simulink model "sampleModel1497"  (R2023a)
settings: Solver=VariableStepAuto  StartTime=0.0  StopTime=10.0  RelTol=1e-3
libraries: hdlsllib x5, simulink x2
settings Model: Creator=user1  LastModifiedBy=user1

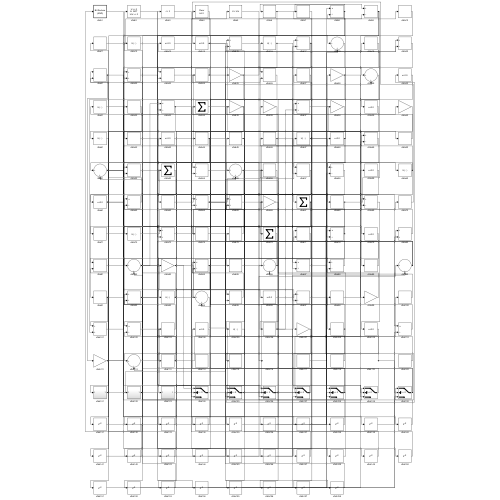
[thumbnail: Simulink's stored preview of the top-level diagram]
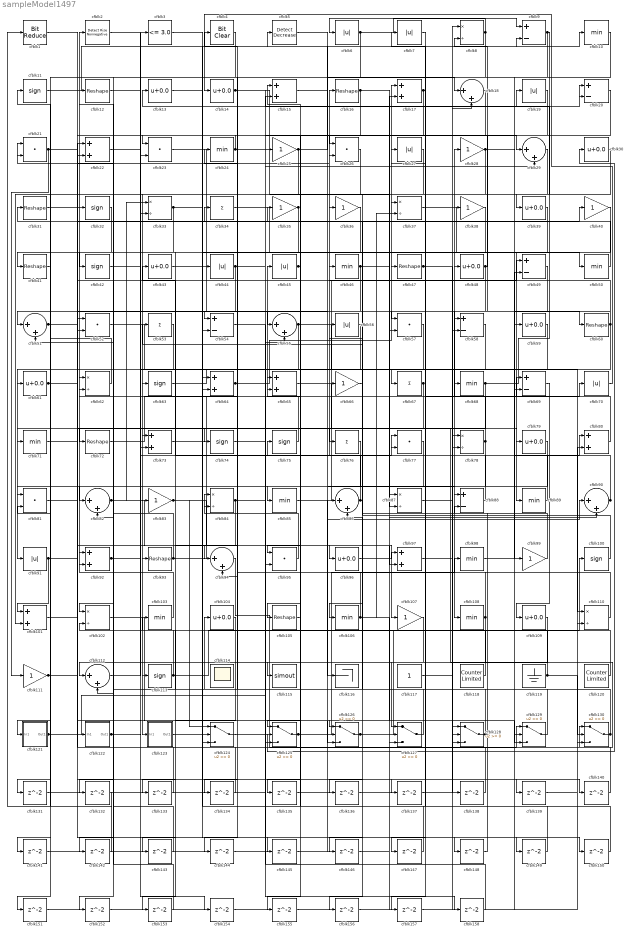
== system sampleModel1497 ==
  cfblk1 : hdlsllib/Logic and Bit Operations/Bit Reduce  mode=AND
  cfblk{10,24,46,50,68,71,85,89,98,103,106,108} (12 alike) : MinMax
  cfblk{11,32,42,63,74..75,100,113} (8 alike) : Signum
  cfblk{15,17,22,64..65,73,80,92,97,101} (10 alike) : Sum
  cfblk{8,33,37,62,78,84,87,102,110} (9 alike) : Product  Inputs=*/  RndMeth=Zero  SaturateOnIntegerOverflow=on
  cfblk{13..14,30,39,43,48,59,61,79,96,104,109} (12 alike) : Bias  Bias=0.0  SaturateOnIntegerOverflow=off
  cfblk{12,16,31,41,47,60,72,93,105} (9 alike) : Reshape
  cfblk{25,28,35..36,38,40,66,83,99,107,111} (11 alike) : Gain
  cfblk{18,29,51,55,82,86,90,94,112} (9 alike) : Sum  Inputs=|++
  cfblk114 : Scope
      settings: Floating=on
  cfblk115 : ToWorkspace  VariableName=simout  SaveFormat=Timeseries  SampleTime=-1
  cfblk116 : Terminator
  cfblk117 : Constant  SampleTime=-1
  cfblk118 : hdlsllib/Sources/Counter Limited  uplimit=7  tsamp=-1
  cfblk119 : Ground
  cfblk120 : hdlsllib/Sources/Counter Limited  uplimit=7  tsamp=-1
  cfblk121 : Subsystem
      settings: LibrarySourceBlock=|
      | hdlsllib/Ports &
      | Subsystems/Subsystem
  cfblk122 : Subsystem
      settings: LibrarySourceBlock=|
      | hdlsllib/Ports &
      | Subsystems/Subsystem
  cfblk123 : Subsystem
      settings: LibrarySourceBlock=|
      | hdlsllib/Ports &
      | Subsystems/Subsystem
  cfblk{124..130} (7 alike) : Switch  SaturateOnIntegerOverflow=off  InputSameDT=off
  cfblk{131..158} (28 alike) : Delay  SampleTime=1
  cfblk{6..7,19,27,44..45,56,70,91} (9 alike) : Abs  SaturateOnIntegerOverflow=off
  cfblk2 : hdlsllib/Logic and Bit Operations/Detect Rise Nonnegative  vinit=0  OutDataTypeStr=boolean
  cfblk{9,20,49,54,58,69,88} (7 alike) : Sum  Inputs=+-
  cfblk{21,23,26,52,57,77,81,95} (8 alike) : DotProduct  OutDataTypeStr=Inherit: Inherit via internal rule
  cfblk3 : hdlsllib/Logic and Bit Operations/Compare To Constant  relop=<=  const=3.0  OutDataTypeStr=boolean
  cfblk{34,53,67,76} (4 alike) : Sum  Inputs=+
  cfblk4 : simulink/Logic and Bit Operations/Bit Clear  iBit=0
      settings: LibrarySourceBlock=|
      | hdlsllib/Logic and Bit
      | Operations/Bit Clear
  cfblk5 : simulink/Logic and Bit Operations/Detect Decrease  vinit=0.0  OutDataTypeStr=boolean
      settings: LibrarySourceBlock=|
      | hdlsllib/Logic and Bit
      | Operations/Detect
      | Decrease
  wires:
  cfblk103/1 -> cfblk2/1
  cfblk82/1 -> cfblk107/1, cfblk128/3, cfblk33/1
  cfblk49/1 -> cfblk108/1
  cfblk83/1 -> cfblk96/1, cfblk124/1
  cfblk106/1 -> cfblk62/1, cfblk129/3, cfblk37/2
  cfblk63/1 -> cfblk67/1
  cfblk53/1 -> cfblk82/1
  cfblk75/1 -> cfblk45/1
  cfblk8/1 -> cfblk6/1, cfblk23/2, cfblk74/1
  cfblk130/1 -> cfblk75/1, cfblk34/1
  cfblk68/1 -> cfblk13/1, cfblk121/1(In1)
  cfblk78/1 -> cfblk28/1, cfblk94/2, cfblk72/1
  cfblk65/1 -> cfblk130/1
  cfblk87/1 -> cfblk128/1
  cfblk48/1 -> cfblk54/1, cfblk8/2
  cfblk94/1 -> cfblk129/1
  cfblk124/1 -> cfblk30/1
  cfblk34/1 -> cfblk89/1
  cfblk1/1 -> cfblk55/1
  cfblk25/1 -> cfblk123/1(In1), cfblk10/1
  cfblk129/1 -> cfblk104/1
  cfblk91/1 -> cfblk101/1, cfblk40/1
  cfblk60/1 -> cfblk51/1, cfblk125/3, cfblk46/1
  cfblk72/1 -> cfblk70/1
  cfblk125/1 -> cfblk98/1, cfblk90/1
  cfblk81/1 -> cfblk49/1
  cfblk85/1 -> cfblk48/1
  cfblk88/1 -> cfblk35/1
  cfblk77/1 -> cfblk93/1
  cfblk64/1 -> cfblk17/1, cfblk126/3, cfblk158/1
  cfblk23/1 -> cfblk116/1
  cfblk119/1 -> cfblk130/2, cfblk12/1
  cfblk28/1 -> cfblk125/1, cfblk60/1
  cfblk61/1 -> cfblk22/1, cfblk124/3
  cfblk86/1 -> cfblk16/1, cfblk56/1
  cfblk7/1 -> cfblk57/1
  cfblk80/1 -> cfblk47/1
  cfblk70/1 -> cfblk14/1
  cfblk89/1 -> cfblk27/1
  cfblk26/1 -> cfblk101/2
  cfblk19/1 -> cfblk58/1
  cfblk126/1 -> cfblk100/1, cfblk90/2
  cfblk96/1 -> cfblk97/1
  cfblk128/1 -> cfblk86/2, cfblk21/1
  cfblk50/1 -> cfblk4/1
  cfblk56/1 -> cfblk63/1
  cfblk67/1 -> cfblk112/1, cfblk95/2
  cfblk93/1 -> cfblk66/1, cfblk51/2
  cfblk47/1 -> cfblk19/1, cfblk129/2
  cfblk5/1 -> cfblk88/1
  cfblk32/1 -> cfblk41/1
  cfblk6/1 -> cfblk9/1, cfblk33/2
  cfblk122/1(Out1) -> cfblk92/1, cfblk154/1
  cfblk90/1 -> cfblk24/1, cfblk7/1, cfblk43/1
  cfblk54/1 -> cfblk79/1
  cfblk92/1 -> cfblk3/1, cfblk124/2, cfblk152/1
  cfblk45/1 -> cfblk85/1, cfblk105/1
  cfblk16/1 -> cfblk57/2, cfblk135/1
  cfblk108/1 -> cfblk31/1, cfblk127/1
  cfblk2/1 -> cfblk68/1
  cfblk9/1 -> cfblk39/1, cfblk22/2, cfblk42/1
  cfblk74/1 -> cfblk69/1
  cfblk69/1 -> cfblk109/1
  cfblk30/1 -> cfblk94/1
  cfblk15/1 -> cfblk18/1
  cfblk123/1(Out1) -> cfblk44/1
  cfblk14/1 -> cfblk87/1, cfblk20/2
  cfblk84/1 -> cfblk29/2, cfblk133/1
  cfblk37/1 -> cfblk99/1
  cfblk59/1 -> cfblk91/1
  cfblk102/1 -> cfblk126/1
  cfblk36/1 -> cfblk113/1
  cfblk21/1 -> cfblk111/1, cfblk73/1
  cfblk98/1 -> cfblk80/1
  cfblk43/1 -> cfblk9/2
  cfblk112/1 -> cfblk77/1
  cfblk10/1 -> cfblk69/2
  cfblk40/1 -> cfblk115/1
  cfblk17/1 -> cfblk102/1, cfblk157/1
  cfblk121/1(Out1) -> cfblk25/1, cfblk21/2
  cfblk73/1 -> cfblk65/1
  cfblk46/1 -> cfblk87/2, cfblk61/1
  cfblk11/1 -> cfblk5/1
  cfblk113/1 -> cfblk82/2, cfblk59/1
  cfblk20/1 -> cfblk26/1
  cfblk62/1 -> cfblk11/1
  cfblk52/1 -> cfblk78/2
  cfblk44/1 -> cfblk20/1, cfblk142/1, cfblk143/1
  cfblk57/1 -> cfblk95/1
  cfblk127/1 -> cfblk103/1
  cfblk76/1 -> cfblk81/1
  cfblk38/1 -> cfblk83/1
  cfblk24/1 -> cfblk23/1, cfblk29/1
  cfblk33/1 -> cfblk71/1, cfblk150/1
  cfblk58/1 -> cfblk106/1
  cfblk120/1 -> cfblk84/1
  cfblk117/1 -> cfblk38/1
  cfblk101/1 -> cfblk32/1
  cfblk12/1 -> cfblk54/2
  cfblk71/1 -> cfblk122/1(In1)
  cfblk3/1 -> cfblk50/1
  cfblk51/1 -> cfblk97/2, cfblk76/1, cfblk137/1
  cfblk18/1 -> cfblk52/2
  cfblk95/1 -> cfblk84/2
  cfblk55/1 -> cfblk110/1, cfblk73/2
  cfblk110/1 -> cfblk15/1
  cfblk35/1 -> cfblk64/2, cfblk131/1
  cfblk111/1 -> cfblk26/2, cfblk145/1
  cfblk100/1 -> cfblk36/1
  cfblk99/1 -> cfblk53/1
  cfblk118/1 -> cfblk37/1
  cfblk131/1 -> cfblk15/2
  cfblk107/1 -> cfblk132/1
  cfblk132/1 -> cfblk1/1
  cfblk133/1 -> cfblk62/2
  cfblk29/1 -> cfblk134/1
  cfblk134/1 -> cfblk52/1
  cfblk135/1 -> cfblk128/2
  cfblk66/1 -> cfblk136/1
  cfblk136/1 -> cfblk78/1
  cfblk137/1 -> cfblk58/2
  cfblk97/1 -> cfblk138/1
  cfblk138/1 -> cfblk112/2
  cfblk31/1 -> cfblk139/1
  cfblk139/1 -> cfblk80/2
  cfblk13/1 -> cfblk140/1
  cfblk140/1 -> cfblk126/2
  cfblk41/1 -> cfblk141/1
  cfblk141/1 -> cfblk55/2
  cfblk142/1 -> cfblk81/2
  cfblk143/1 -> cfblk102/2
  cfblk109/1 -> cfblk144/1
  cfblk144/1 -> cfblk86/1
  cfblk145/1 -> cfblk127/3
  cfblk79/1 -> cfblk146/1
  cfblk146/1 -> cfblk17/2
  cfblk39/1 -> cfblk147/1
  cfblk147/1 -> cfblk65/2
  cfblk22/1 -> cfblk148/1
  cfblk148/1 -> cfblk88/2
  cfblk42/1 -> cfblk149/1
  cfblk149/1 -> cfblk77/2
  cfblk150/1 -> cfblk64/1
  cfblk4/1 -> cfblk151/1
  cfblk151/1 -> cfblk110/2
  cfblk152/1 -> cfblk8/1
  cfblk104/1 -> cfblk153/1
  cfblk153/1 -> cfblk92/2
  cfblk154/1 -> cfblk127/2
  cfblk105/1 -> cfblk155/1
  cfblk155/1 -> cfblk49/2
  cfblk27/1 -> cfblk156/1
  cfblk156/1 -> cfblk130/3
  cfblk157/1 -> cfblk18/2
  cfblk158/1 -> cfblk125/2

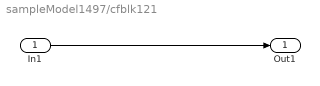
== system sampleModel1497/cfblk121 ==
  In1 : Inport
  Out1 : Outport
  wires:
  In1/1 -> Out1/1

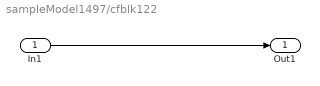
== system sampleModel1497/cfblk122 ==
  In1 : Inport
  Out1 : Outport
  wires:
  In1/1 -> Out1/1

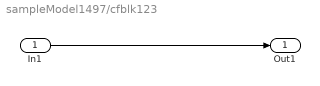
== system sampleModel1497/cfblk123 ==
  In1 : Inport
  Out1 : Outport
  wires:
  In1/1 -> Out1/1
